simulink model "MassaMollaSmorzatore"  (R2019b)
settings: Solver=VariableStepAuto  StartTime=0.0  StopTime=10.0  MaxStep=1e-4  RelTol=1e-3
values from neighbouring files (symbols this model uses):
  A = [0 , 1; 0 , -(bb/(Mi*Ei*Ei+Ie))-(( (Ud*Mi*Ei*Ei)/(Mi*Ei*Ei+Ie) )*2*We) ]    [Progetto3a.m]    (also in Progetto4c.m = [0, 1; ((-gg*mm*ee)*cos(pi/2))/((mm*ee*ee+Ie)), -beta/(mm*ee; ProgettoGruppoAO.m; Progetto_Ada.m = [0, 1; ((-gg*mm*ee)*cos(pi/2))/((mm*ee*ee+Ie)), -beta/(mm*ee; Prova.m = [0, 1; 0, (bb/(Mi*Ei*Ei+Ie))-(( (Ud*Mi*Ei*Ei)/(Mi*Ei*Ei+Ie) )
  B = [0; 1/(Mi*Ei*Ei+Ie)]    [Progetto3a.m]    (also in Progetto4c.m = [0;1/(mm*ee*ee + Ie)]; ProgettoGruppoAO.m; Progetto_Ada.m = [0;1/(mm*ee*ee + Ie)]; Prova.m)
  beta = 0.3    [Progetto4c.m]    (also in Progetto_Ada.m)
  C = [0 , 1]    [Progetto3a.m]    (also in Progetto4c.m = [0, 1]; ProgettoGruppoAO.m; Progetto_Ada.m = [0, 1]; Prova.m = [0, 1])
  den_r = d_r{1}    [Progetto3a.m]    (also in Progetto4c.m; ProgettoGruppoAO.m; Progetto_Ada.m; Prova.m)
  mm = 0.15    [Progetto4c.m]    (also in Progetto_Ada.m)
  num_r = n_r{1}    [Progetto3a.m]    (also in Progetto4c.m; ProgettoGruppoAO.m; Progetto_Ada.m; Prova.m)
  omega_n = 100    [Progetto3a.m]    (also in Progetto4c.m = 120; ProgettoGruppoAO.m; Progetto_Ada.m = 120; Prova.m)
  W = 5    [Progetto3a.m]    (also in Progetto4c.m = 4; ProgettoGruppoAO.m; Progetto_Ada.m = 4; Prova.m)
  x0 = [0,We]    [Progetto3a.m]    (also in Progetto4c.m = [0;0]; ProgettoGruppoAO.m = [teta_e,We]; Progetto_Ada.m = [0;0]; Prova.m = [teta_e,We])
undefined symbols (not defined in the file or in its folder): kk
settings Model: Creator=spiri  LastModifiedBy=spiri

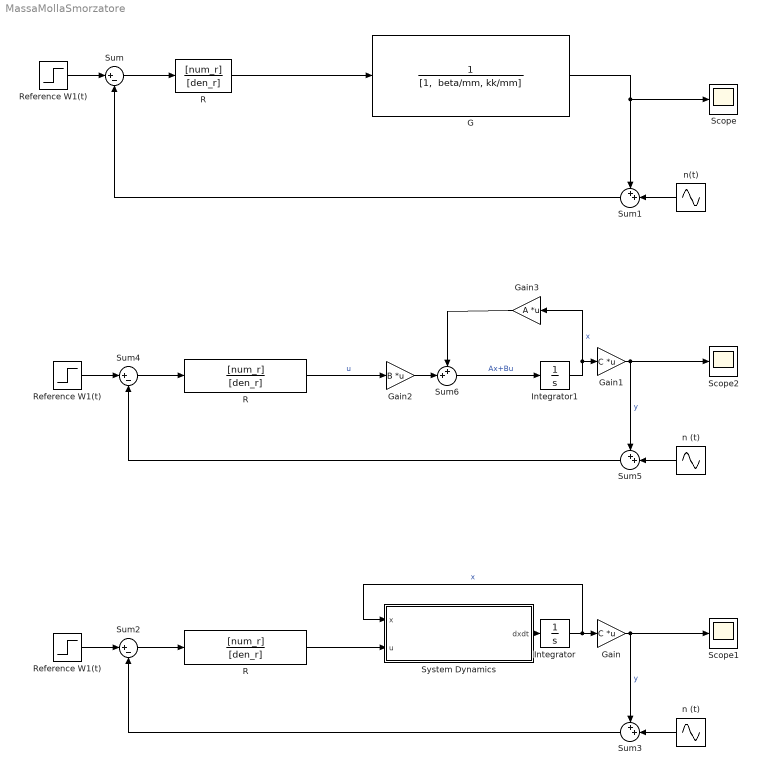
== system MassaMollaSmorzatore ==
  G : TransferFcn  Denominator="[1,  beta/mm, kk/mm]"
  Gain : Gain  Gain=C  Multiplication=Matrix(K*u)
  Gain1 : Gain  Gain=C  Multiplication=Matrix(K*u)
  Gain2 : Gain  Gain=B  Multiplication=Matrix(K*u)
  Gain3 : Gain  Gain=A  Multiplication=Matrix(K*u)
  Integrator : Integrator  InitialCondition=x0
  Integrator1 : Integrator  InitialCondition=x0
  R : TransferFcn  Numerator=[num_r]  Denominator=[den_r]
  "R " : TransferFcn  Numerator=[num_r]  Denominator=[den_r]
  "R " : TransferFcn  Numerator=[num_r]  Denominator=[den_r]
  Reference W1(t) : Step  After=W  SampleTime=0
  "Reference W1(t) " : Step  After=W  SampleTime=0
  "Reference W1(t) " : Step  After=W  SampleTime=0
  Scope : Scope
  Scope1 : Scope
  Scope2 : Scope
  Sum : Sum  Inputs=|+-
  Sum{1,3,5..6} (4 alike) : Sum  Inputs=++|
  Sum2 : Sum  Inputs=|+-
  Sum4 : Sum  Inputs=|+-
  System Dynamics : MATLAB Function  TreatAsAtomicUnit=on
  n (t) : Sin  Amplitude=0.01  Frequency=omega_n  SampleTime=0
  "n (t) " : Sin  Amplitude=0.01  Frequency=omega_n  SampleTime=0
  n(t) : Sin  Amplitude=0.01  Frequency=omega_n  SampleTime=0
  wires:
  n(t)/1 -> Sum1/2
  Sum1/1 -> Sum/2
  Reference W1(t)/1 -> Sum/1
  G/1 -> Scope/1, Sum1/1
  Sum/1 -> R/1
  R/1 -> G/1
  "R "/1 -> System Dynamics/2(u)
  Sum2/1 -> "R "/1
  "Reference W1(t) "/1 -> Sum2/1
  Sum3/1 -> Sum2/2
  n (t)/1 -> Sum3/2
  System Dynamics/1(dxdt) -> Integrator/1
  Integrator/1 -> System Dynamics/1(x), Gain/1  "x"
  Gain/1 -> Scope1/1, Sum3/1  "y"
  Gain1/1 -> Sum5/1, Scope2/1  "y"
  Integrator1/1 -> Gain1/1, Gain3/1  "x"
  Sum6/1 -> Integrator1/1  "Ax+Bu"
  "n (t) "/1 -> Sum5/2
  Sum5/1 -> Sum4/2
  "Reference W1(t) "/1 -> Sum4/1
  Sum4/1 -> "R "/1
  "R "/1 -> Gain2/1  "u"
  Gain2/1 -> Sum6/2
  Gain3/1 -> Sum6/1

== matlab function MassaMollaSmorzatore/System Dynamics ==
  data: x input; u input; dxdt output
function dxdt = systemDynamics(x,u)
mm=0.5; %[kg] Mass
beta=0.3; %[N/m^2] Dynamic Friction coefficient
kk=1; % [N/m] Spring stiffness constant

dx1dt=x(2);
dx2dt=(-kk*x(1)- beta*x(2) + u)/mm;
%dxdt = [dx1dt; dx2dt; dx3dt;...;dxndt];
dxdt = [dx1dt; dx2dt;];
